simulink model "Funcion"  (R2017b)
settings: Solver=ode23t  StartTime=0.0  StopTime=10000  RelTol=1e-3
undefined symbols (not defined in the file): AH, AH0, AH1, B1, B2, B3, Ri, V1, Vnom
libraries: nesl_utility x9, fl_lib x8, elec_lib x6
settings Model: Creator=maxed  LastModifiedBy=maxed
settings SolverCC: AlgebraicLoopSolver=LineSearch

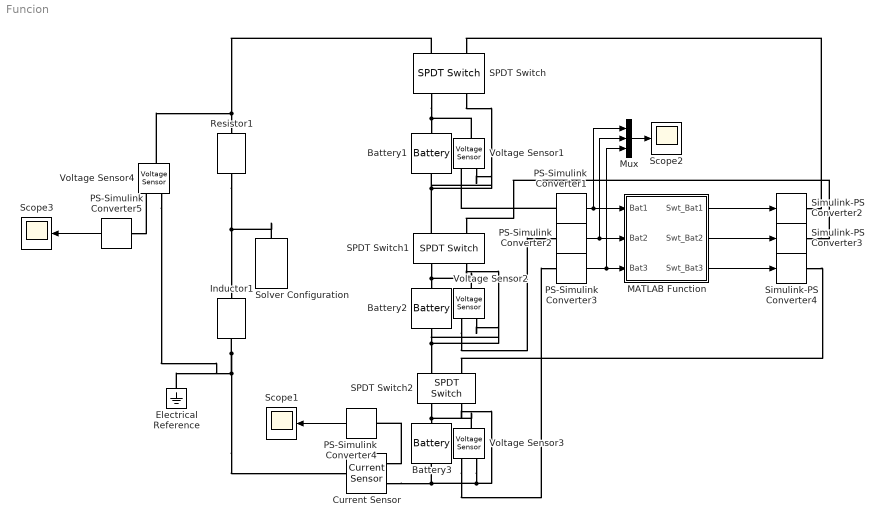
== system Funcion ==
  Battery1 : elec_lib/Sources/Battery  Vnom=B1*Vnom V  R1=B1*Ri Ohm  prm_AH=2  AH=B1*AH hr*A  V1=B1*V1 V  AH1=B1*AH1 hr*A  prm_R2=1  R2=2000 Ohm  prm_fade=1  N_fade=100  AH_fade=45 hr*A  R1_fade=2.02 Ohm  V1_fade=10.35 V  i_specify=off  i_priority=None  i=0 A  i_nominal_specify=off  i_nominal_unit=A  i_nominal_value=1  v_specify=off  v_priority=None  v=0 V  v_nominal_specify=off  v_nominal_unit=V  v_nominal_value=1  charge_specify=on  charge_priority=High  charge=B1*AH0 hr*A  charge_nominal_specify=off  charge_nominal_unit=hr*A  charge_nominal_value=1  num_cycles_specify=off  num_cycles_priority=High  num_cycles=0  num_cycles_nominal_specify=off  num_cycles_nominal_unit=1  num_cycles_nominal_value=1  thermal_mass=30000 J/K  Tmeas=298.15 K  Vnom_T2=12 V  R1_T2=2.2 Ohm  V1_T2=11.4 V  R2_T2=2200 Ohm  Tmeas2=273.15 K  temperature_specify=off  temperature_priority=High  temperature=298.15 K  temperature_nominal_specify=off  temperature_nominal_unit=K  temperature_nominal_value=1
      settings: SourceProductName=Simscape Electronics  SourceProductBaseCode=SN
  Battery2 : elec_lib/Sources/Battery  Vnom=B2*Vnom V  R1=Ri Ohm  prm_AH=2  AH=B2*AH hr*A  V1=B2*V1 V  AH1=B2*AH1 hr*A  prm_R2=1  R2=2000 Ohm  prm_fade=1  N_fade=100  AH_fade=45 hr*A  R1_fade=2.02 Ohm  V1_fade=10.35 V  i_specify=off  i_priority=None  i=0 A  i_nominal_specify=off  i_nominal_unit=A  i_nominal_value=1  v_specify=off  v_priority=None  v=0 V  v_nominal_specify=off  v_nominal_unit=V  v_nominal_value=1  charge_specify=on  charge_priority=High  charge=B2*AH0 hr*A  charge_nominal_specify=off  charge_nominal_unit=hr*A  charge_nominal_value=1  num_cycles_specify=off  num_cycles_priority=High  num_cycles=0  num_cycles_nominal_specify=off  num_cycles_nominal_unit=1  num_cycles_nominal_value=1  thermal_mass=30000 J/K  Tmeas=298.15 K  Vnom_T2=12 V  R1_T2=2.2 Ohm  V1_T2=11.4 V  R2_T2=2200 Ohm  Tmeas2=273.15 K  temperature_specify=off  temperature_priority=High  temperature=298.15 K  temperature_nominal_specify=off  temperature_nominal_unit=K  temperature_nominal_value=1
      settings: SourceProductName=Simscape Electronics  SourceProductBaseCode=SN
  Battery3 : elec_lib/Sources/Battery  Vnom=B3*Vnom V  R1=B3*Ri Ohm  prm_AH=2  AH=B3*AH hr*A  V1=B3*V1 V  AH1=B3*AH1 hr*A  prm_R2=1  R2=2000 Ohm  prm_fade=1  N_fade=100  AH_fade=45 hr*A  R1_fade=2.02 Ohm  V1_fade=10.35 V  i_specify=off  i_priority=None  i=0 A  i_nominal_specify=off  i_nominal_unit=A  i_nominal_value=1  v_specify=off  v_priority=None  v=0 V  v_nominal_specify=off  v_nominal_unit=V  v_nominal_value=1  charge_specify=on  charge_priority=High  charge=B3*AH0 hr*A  charge_nominal_specify=off  charge_nominal_unit=hr*A  charge_nominal_value=1  num_cycles_specify=off  num_cycles_priority=High  num_cycles=0  num_cycles_nominal_specify=off  num_cycles_nominal_unit=1  num_cycles_nominal_value=1  thermal_mass=30000 J/K  Tmeas=298.15 K  Vnom_T2=12 V  R1_T2=2.2 Ohm  V1_T2=11.4 V  R2_T2=2200 Ohm  Tmeas2=273.15 K  temperature_specify=off  temperature_priority=High  temperature=298.15 K  temperature_nominal_specify=off  temperature_nominal_unit=K  temperature_nominal_value=1
      settings: SourceProductName=Simscape Electronics  SourceProductBaseCode=SN
  Current Sensor : fl_lib/Electrical/Electrical Sensors/Current Sensor
  Electrical Reference : fl_lib/Electrical/Electrical Elements/Electrical Reference
  Inductor1 : fl_lib/Electrical/Electrical Elements/Inductor  l=10 mH  r=0 Ohm  g=1e-9 1/Ohm  i_specify=off  i_priority=None  i=0 A  i_nominal_specify=off  i_nominal_unit=A  i_nominal_value=1  v_specify=off  v_priority=None  v=0 V  v_nominal_specify=off  v_nominal_unit=V  v_nominal_value=1  i_L_specify=off  i_L_priority=High  i_L=0 A  i_L_nominal_specify=off  i_L_nominal_unit=A  i_L_nominal_value=1
  MATLAB Function : MATLAB Function  TreatAsAtomicUnit=on
  Mux : Mux  Inputs=3
  PS-Simulink Converter{1..5} (5 alike) : nesl_utility/PS-Simulink Converter  PhysicalDomain=network_engine_domain  SubClassName=ps_output  LeftPortType=input  RightPortType=output  PseudoPeriodic=off  Frequencies=[]  Unit=1  AffineConversion=off
  Resistor1 : fl_lib/Electrical/Electrical Elements/Resistor  R=50 Ohm  i_specify=off  i_priority=None  i=0 A  i_nominal_specify=off  i_nominal_unit=A  i_nominal_value=1  v_specify=off  v_priority=None  v=0 V  v_nominal_specify=off  v_nominal_unit=V  v_nominal_value=1
  SPDT Switch : elec_lib/Passive Devices/Switches/SPDT Switch  R_closed=0.01 Ohm  G_open=1e-6 S  Threshold=0 V  Width=0 V  model_dynamics=0  t_on=1e-3 s  t_off=1e-3 s  initial_vT=0 V
      settings: SourceProductName=Simscape Electronics  SourceProductBaseCode=SN
  SPDT Switch1 : elec_lib/Passive Devices/Switches/SPDT Switch  R_closed=0.01 Ohm  G_open=1e-6 S  Threshold=0 V  Width=0 V  model_dynamics=0  t_on=1e-3 s  t_off=1e-3 s  initial_vT=0 V
      settings: SourceProductName=Simscape Electronics  SourceProductBaseCode=SN
  SPDT Switch2 : elec_lib/Passive Devices/Switches/SPDT Switch  R_closed=0.01 Ohm  G_open=1e-6 S  Threshold=0 V  Width=0 V  model_dynamics=0  t_on=1e-3 s  t_off=1e-3 s  initial_vT=0 V
      settings: SourceProductName=Simscape Electronics  SourceProductBaseCode=SN
  Scope1 : Scope
  Scope2 : Scope
  Scope3 : Scope
  Simulink-PS Converter2 : nesl_utility/Simulink-PS Converter  PhysicalDomain=network_engine_domain  SubClassName=ps_input  LeftPortType=input  RightPortType=output  PseudoPeriodic=off  Frequencies=[]  NoiseDistribution=none  NoiseParameters=[]  Unit=1  AffineConversion=off  FilteringAndDerivatives=provide  SimscapeFilterOrder=1  InputFilterTimeConstant=0.001  UdotUserProvided=0
  Simulink-PS Converter3 : nesl_utility/Simulink-PS Converter  PhysicalDomain=network_engine_domain  SubClassName=ps_input  LeftPortType=input  RightPortType=output  PseudoPeriodic=off  Frequencies=[]  NoiseDistribution=none  NoiseParameters=[]  Unit=1  AffineConversion=off  FilteringAndDerivatives=provide  SimscapeFilterOrder=1  InputFilterTimeConstant=0.001  UdotUserProvided=0
  Simulink-PS Converter4 : nesl_utility/Simulink-PS Converter  PhysicalDomain=network_engine_domain  SubClassName=ps_input  LeftPortType=input  RightPortType=output  PseudoPeriodic=off  Frequencies=[]  NoiseDistribution=none  NoiseParameters=[]  Unit=1  AffineConversion=off  FilteringAndDerivatives=provide  SimscapeFilterOrder=1  InputFilterTimeConstant=0.001  UdotUserProvided=0
  Solver Configuration : nesl_utility/Solver Configuration  PhysicalDomain=network_engine_domain  SubClassName=solver  LeftPortType=input  RightPortType=generic  Accelerate=off  Tones=[]  Harmonics=[]  SimulateNoise=off  Profile=off  UseLocalSampling=off  EnableSwitchedLinearOptims=on  FrequencyDomain=off  UseCCode=off  RelTol=0.001  AbsTol=1e-06  MinStep=1e-09  ToWorkspace=off  RevertToSquareIcSolve=off  NumHomotopyIterations=100  PhasorMode=off  PhasorModeNumHarmonics=1  DoDC=on  ResidualTolerance=1e-09  UseLocalSolver=on  LocalSolverChoice=NE_BACKWARD_EULER_ADVANCER  LocalSolverSampleTime=Ts  DoFixedCost=on  MaxNonlinIter=3  MaxModeIter=2  LinearAlgebra=Sparse  DelaysMemoryBudget=1024  AutomaticFiltering=on  FilteringTimeConstant=0.001
  Voltage Sensor{1..4} (4 alike) : fl_lib/Electrical/Electrical Sensors/Voltage Sensor
  wires:
  PS-Simulink Converter1/1 -> Mux/1, MATLAB Function/1(Bat1)
  PS-Simulink Converter2/1 -> Mux/2, MATLAB Function/2(Bat2)
  PS-Simulink Converter3/1 -> Mux/3, MATLAB Function/3(Bat3)
  MATLAB Function/1(Swt_Bat1) -> Simulink-PS Converter2/1
  MATLAB Function/2(Swt_Bat2) -> Simulink-PS Converter3/1
  MATLAB Function/3(Swt_Bat3) -> Simulink-PS Converter4/1
  PS-Simulink Converter4/1 -> Scope1/1
  Mux/1 -> Scope2/1
  PS-Simulink Converter5/1 -> Scope3/1
  connections:
  SPDT Switch/RConn2 -- Voltage Sensor1/LConn1 -- Battery1/LConn1
  SPDT Switch1/LConn2 -- Voltage Sensor1/RConn2 -- SPDT Switch/RConn1 -- Battery1/RConn1
  SPDT Switch1/RConn2 -- Voltage Sensor2/LConn1 -- Battery2/LConn1
  Battery2/RConn1 -- Voltage Sensor2/RConn2 -- SPDT Switch1/RConn1 -- SPDT Switch2/LConn2
  SPDT Switch2/RConn2 -- Voltage Sensor3/LConn1 -- Battery3/LConn1
  Voltage Sensor3/RConn2 -- SPDT Switch2/RConn1 -- Current Sensor/RConn2 -- Battery3/RConn1
  PS-Simulink Converter1/LConn1 -- Voltage Sensor1/RConn1
  Voltage Sensor2/RConn1 -- PS-Simulink Converter2/LConn1
  Voltage Sensor3/RConn1 -- PS-Simulink Converter3/LConn1
  Simulink-PS Converter4/RConn1 -- SPDT Switch2/LConn1
  Simulink-PS Converter3/RConn1 -- SPDT Switch1/LConn1
  Simulink-PS Converter2/RConn1 -- SPDT Switch/LConn1
  SPDT Switch/LConn2 -- Voltage Sensor4/LConn1 -- Resistor1/LConn1
  Resistor1/RConn1 -- Solver Configuration/RConn1 -- Inductor1/LConn1
  Inductor1/RConn1 -- Voltage Sensor4/RConn2 -- Electrical Reference/LConn1 -- Current Sensor/LConn1
  Current Sensor/RConn1 -- PS-Simulink Converter4/LConn1
  PS-Simulink Converter5/LConn1 -- Voltage Sensor4/RConn1

== matlab function Funcion/MATLAB Function ==
  data: Swt_Bat1 output; Bat1 input; Swt_Bat2 output; Bat2 input; Bat3 input; Swt_Bat3 output
function [Swt_Bat1, Swt_Bat2, Swt_Bat3]= fcn(Bat1, Bat2, Bat3)
Bat1_vol_init = Bat1;
Bat2_vol_init = Bat2;
Bat3_vol_init = Bat3;
while (1)
    if Bat1 > Bat1_vol_init*0.80
        Swt_Bat1=1;
    else
        Swt_Bat1=0;
    end
    if Bat2 > Bat2_vol_init*0.80
        Swt_Bat2=1;
    else
        Swt_Bat2=0;
    end
    if Bat3 > Bat3_vol_init*0.80
        Swt_Bat3=1;
    else
        Swt_Bat3=0;
    end
end
